simulink model "circonvsimulink"  (R2022b)
settings: Solver=VariableStepAuto  StartTime=0.0  StopTime=0  RelTol=1e-3
settings Model: Creator=DSP-27  LastModifiedBy=DSP-27

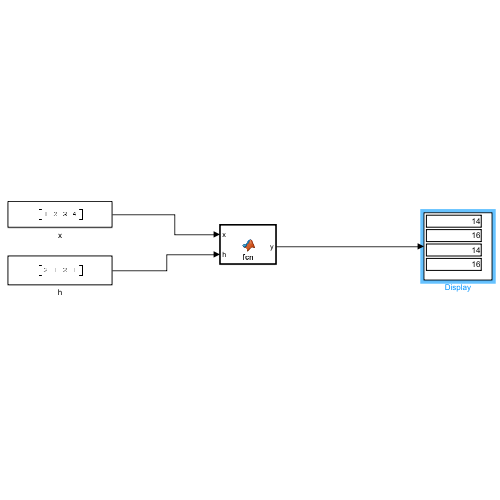
[thumbnail: Simulink's stored preview of the top-level diagram]
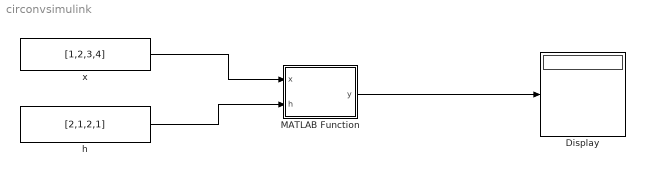
== system circonvsimulink ==
  Display : Display
  MATLAB Function : MATLAB Function  TreatAsAtomicUnit=on
  h : Constant  Value=[2,1,2,1]
  x : Constant  Value=[1,2,3,4]
  wires:
  MATLAB Function/1(y) -> Display/1
  h/1 -> MATLAB Function/2(h)
  x/1 -> MATLAB Function/1(x)

== matlab function circonvsimulink/MATLAB Function ==
  data: y output; x input; h input

function y = fcn(x,h)

m = length(h);
n = length(x);
num = 0;
max_len = max(n, m);
    H = zeros(max_len, max_len);

    for i = 1:max_len
        if i == 1
           H(:,i) = h(:);
           num = H(max_len, i);
        else
            H(1,i) = num;
            H(2:max_len, i) = H(1:max_len-1, i-1);
            num = H(max_len, i);
        end
    end
    y = H*x;
end
